simulink model "StateSpaceSystem"  (R2018b)
settings: Solver=VariableStepAuto  StartTime=0.0  StopTime=10.0  RelTol=1e-3
settings Model: Creator=Seko  LastModifiedBy=Seko

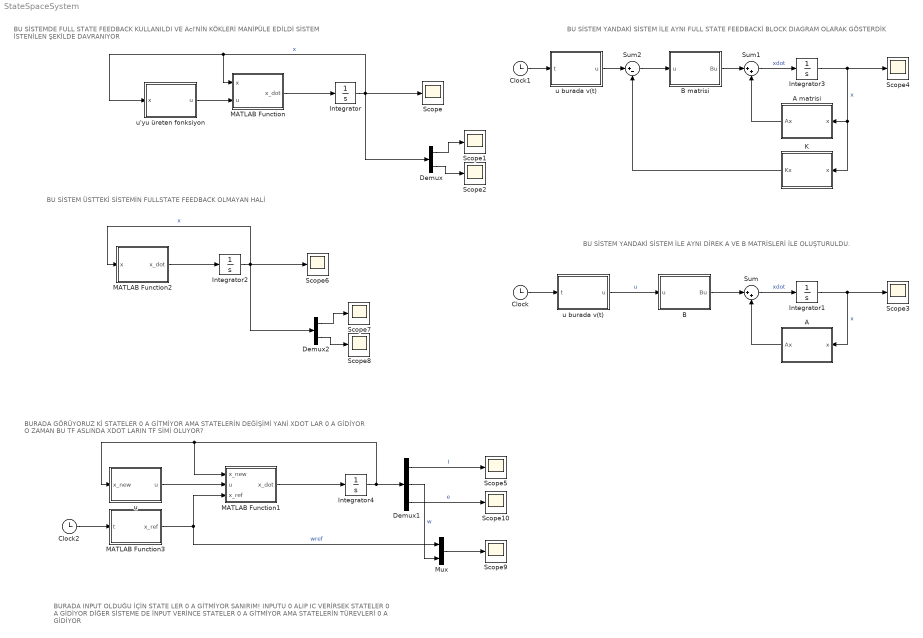
== system StateSpaceSystem ==
  note: BURADA GÖRÜYORUZ Kİ STATELER 0 A GİTMİYOR AMA STATELERİN DEĞİŞİMİ YANİ XDOT LAR 0 A GİDİYOR O ZAMAN BU TF ASLINDA XDOT LARIN TF SİMİ OLUYOR?
  note: BU SİSTEM YANDAKİ SİSTEM İLE AYNI DİREK A VE B MATRİSLERİ İLE OLUŞTURULDU.
  note: BU SİSTEMDE FULL STATE FEEDBACK KULLANILDI VE Acl'NİN KÖKLERİ MANİPÜLE EDİLDİ SİSTEM İSTENİLEN ŞEKİLDE DAVRANIYOR
  note: BU SİSTEM ÜSTTEKİ SİSTEMİN FULLSTATE FEEDBACK OLMAYAN HALİ
  note: BU SİSTEM YANDAKİ SİSTEM İLE AYNI FULL STATE FEEDBACKİ BLOCK DIAGRAM OLARAK GÖSTERDİK
  note: BURADA INPUT OLDUĞU İÇİN STATE LER 0 A GİTMİYOR SANIRIM! INPUTU 0 ALIP IC VERİRSEK STATELER 0 A GİDİYOR
      |
      | DİĞER SİSTEME DE İNPUT VERİNCE STATELER 0 A GİTMİYOR AMA STATELERİN TÜREVLERİ 0 A GİDİYOR
  A : MATLAB Function  TreatAsAtomicUnit=on
  A matrisi : MATLAB Function  TreatAsAtomicUnit=on
  B : MATLAB Function  TreatAsAtomicUnit=on
  B matrisi : MATLAB Function  TreatAsAtomicUnit=on
  Clock : Clock
  Clock1 : Clock
  Clock2 : Clock
  Demux : Demux  Outputs=2
  Demux1 : Demux  Outputs=3
  Demux2 : Demux  Outputs=2
  Integrator{,1..3} (4 alike) : Integrator  InitialCondition=[100;20]
  Integrator4 : Integrator  InitialCondition=[10;10;10]
  K : MATLAB Function  TreatAsAtomicUnit=on
  MATLAB Function : MATLAB Function  TreatAsAtomicUnit=on
  MATLAB Function1 : MATLAB Function  TreatAsAtomicUnit=on
  MATLAB Function2 : MATLAB Function  TreatAsAtomicUnit=on
  MATLAB Function3 : MATLAB Function  TreatAsAtomicUnit=on
  Mux : Mux  Inputs=2
  Scope{,1..10} (11 alike) : Scope
  Sum : Sum  Inputs=|++
  Sum1 : Sum  Inputs=|++
  Sum2 : Sum  Inputs=|+-
  u : MATLAB Function  TreatAsAtomicUnit=on
  u burada v(t) : MATLAB Function  TreatAsAtomicUnit=on
  "u burada v(t) " : MATLAB Function  TreatAsAtomicUnit=on
  "u'yu üreten fonksiyon " : MATLAB Function  TreatAsAtomicUnit=on
  wires:
  MATLAB Function/1(x_dot) -> Integrator/1
  Integrator/1 -> Demux/1, Scope/1, MATLAB Function/1(x), "u'yu üreten fonksiyon "/1(x)  "x"
  "u'yu üreten fonksiyon "/1(u) -> MATLAB Function/2(u)
  Demux/1 -> Scope1/1
  Demux/2 -> Scope2/1
  Demux2/2 -> Scope8/1
  Demux2/1 -> Scope7/1
  Integrator2/1 -> Demux2/1, Scope6/1, MATLAB Function2/1(x)  "x"
  MATLAB Function2/1(x_dot) -> Integrator2/1
  B/1(Bu) -> Sum/1
  Sum/1 -> Integrator1/1  "xdot"
  Integrator1/1 -> Scope3/1, A/1(x)  "x"
  A/1(Ax) -> Sum/2
  Clock/1 -> "u burada v(t) "/1(t)
  "u burada v(t) "/1(u) -> B/1(u)  "u"
  Clock1/1 -> u burada v(t)/1(t)
  Integrator3/1 -> Scope4/1, K/1(x), A matrisi/1(x)  "x"
  B matrisi/1(Bu) -> Sum1/1
  Sum1/1 -> Integrator3/1  "xdot"
  A matrisi/1(Ax) -> Sum1/2
  K/1(Kx) -> Sum2/2
  Sum2/1 -> B matrisi/1(u)
  u burada v(t)/1(u) -> Sum2/1
  MATLAB Function1/1(x_dot) -> Integrator4/1
  Integrator4/1 -> Demux1/1, MATLAB Function1/1(x_new), u/1(x_new)
  u/1(u) -> MATLAB Function1/2(u)
  Clock2/1 -> MATLAB Function3/1(t)
  MATLAB Function3/1(x_ref) -> MATLAB Function1/3(x_ref), Mux/1  "wref"
  Mux/1 -> Scope9/1
  Demux1/2 -> Mux/2  "w"
  Demux1/1 -> Scope5/1  "I"
  Demux1/3 -> Scope10/1  "e"

== matlab function StateSpaceSystem/u'yu üreten fonksiyon  ==
  data: x input; u output
function u = fcn(x)
K=[-0.3389    0.3913]; % Bu değerleri place fonksiyonundan bulduk.
u = -K*x; 
end

== matlab function StateSpaceSystem/MATLAB Function ==
  data: x input; u input; x_dot output
function x_dot = fcn(x,u)
%% Motor sistemi için A ve B state space matrislerini oluşturulaım:
%Real parameter values:
R=0.55;
Kt=85*10^-3;
L=25*10^-3;
J=0.06+0.03;
b=0.05;

%State space matrix (Bunu video 21'de çıkardık)
a00=-R/L;
a01=-Kt/L;
a10= Kt/J;
a11= -b/J;

b00=1/L;
b10=0;

A=[a00,a11;
   a10,a11];

B=[b00; 
    b10];
%%
%% Sistemin State Space Denklemi'ni yazıyoruz:
x_dot=A*x+B*u;

end

== matlab function StateSpaceSystem/B ==
  data: u input; Bu output
function Bu = fcn(u)

%B matrisini tanımlıyoruz
L=25*10^-3;

b00=1/L;
b10=0;

B=[b00; 
   b10];
%B*x i tanımlıyoruz
Bu=B*u;

end

== matlab function StateSpaceSystem/A ==
  data: x input; Ax output
function Ax = fcn(x)

R=0.55;
Kt=85*10^-3;
L=25*10^-3;
J=0.06+0.03;
b=0.05;

a00=-R/L;
a01=-Kt/L;
a10= Kt/J;
a11= -b/J;

A=[a00,a11;
   a10,a11];
Ax= A*x;
end

== matlab function StateSpaceSystem/MATLAB Function2 ==
  data: x input; x_dot output
function x_dot = fcn(x)
%% Motor sistemi için A ve B state space matrislerini oluşturulaım:
%Real parameter values:
R=0.55;
Kt=85*10^-3;
L=25*10^-3;
J=0.06+0.03;
b=0.05;

%State space matrix (Bunu video 21'de çıkardık)
a00=-R/L;
a01=-Kt/L;
a10= Kt/J;
a11= -b/J;

b00=1/L;
b10=0;

A=[a00,a11;
   a10,a11];

B=[b00; 
    b10];
%%
%% Sistemin State Space Denklemi'ni yazıyoruz:
x_dot=A*x;

end

== matlab function StateSpaceSystem/u burada v(t)  ==
  data: t input; u output
function u = fcn(t)
u=0*t;
end

== matlab function StateSpaceSystem/A matrisi ==
  data: x input; Ax output
function Ax = fcn(x)

R=0.55;
Kt=85*10^-3;
L=25*10^-3;
J=0.06+0.03;
b=0.05;

a00=-R/L;
a01=-Kt/L;
a10= Kt/J;
a11= -b/J;

A=[a00,a11;
   a10,a11];
Ax= A*x;
end

== matlab function StateSpaceSystem/B matrisi ==
  data: u input; Bu output
function Bu = fcn(u)

%B matrisini tanımlıyoruz
L=25*10^-3;

b00=1/L;
b10=0;

B=[b00; 
   b10];
%B*x i tanımlıyoruz
Bu=B*u;

end

== matlab function StateSpaceSystem/u burada v(t) ==
  data: t input; u output
function u = fcn(t)
u=0*t;

end

== matlab function StateSpaceSystem/K ==
  data: x input; Kx output
function Kx = fcn(x)
K=[-0.3389    0.3913]; % Bu değerleri place fonksiyonundan bulduk.
Kx = K*x; 
end

== matlab function StateSpaceSystem/MATLAB Function1 ==
  data: x_new input; u input; x_dot output; x_ref input
function x_dot = fcn(x_new,u,x_ref)
%% Önce eski A ve B yi tanımlıyorum ki oradan Anew Bnew tanımlanacak
%Real parameter values:
R=0.55;
Kt=85*10^-3;
L=25*10^-3;
J=0.06+0.03;
b=0.05;

%State space matrix (Bunu video 21'de çıkardık)
a00=-R/L;
a01=-Kt/L;
a10= Kt/J;
a11= -b/J;

b00=1/L;
b10=0;

A=[a00,a11;
   a10,a11];

B=[b00; 
    b10];
%%
%% Anew ve Bnew Eref tanımlanıyor

A_new = [A, zeros(2,1);
         0, 1, 0];
B_new = [B;
         0];
E_ref = [0;
         0;
         -1];
%%

%% Şimdi xdot tanımlanıyor. Yani yeni state space equation'ı.

x_dot=A_new*x_new+B_new*u+E_ref*x_ref
end

== matlab function StateSpaceSystem/u ==
  data: x_new input; u output
function u = fcn(x_new)
K=[0.7361   21.9943  116.4706]; %Bunu place komutundan bulduk. İstenen p köklerini tanımladıktan sonra bize gerekli K matrisini matlab vermişti.
u=-K*x_new;
end

== matlab function StateSpaceSystem/MATLAB Function3 ==
  data: t input; x_ref output
function x_ref = fcn(t)

%Burada x_ref dediğimiz w_ref olmuş oluyor çünkü A matrisini öyle seçtik.
bias=50;
A=0;
f=0.1;

x_ref=bias+A*sin(2*pi*f*t);
%x_ref=0;

end
